simulink model "TRQCTL"  (R2022b)
settings: configuration reference "SharedConfig" (kept outside this file)
values from neighbouring files (symbols this model uses):
  MotTqCon_C = 0.054    [TRQCTL.sldd]
  MotTqGainBdT1_Ax : value not decoded    [TRQCTL.sldd]
  MotTqGainBdT1_T : value not decoded    [TRQCTL.sldd]
  MotTqGainBdT2_Ax : value not decoded    [TRQCTL.sldd]
  MotTqGainBdT2_T : value not decoded    [TRQCTL.sldd]
  MotTqMaxDialEna_C = 0.0    [TRQCTL.sldd]
  MotTqMaxDialVal_C = 0.0    [TRQCTL.sldd]
  MotTqMaxMotSpd_Ax : value not decoded    [TRQCTL.sldd]
  MotTqMaxMotSpd_T : value not decoded    [TRQCTL.sldd]
  PhaCurDTarVal_C = 0.0    [TRQCTL.sldd]
  PhaCurQTarDialEna_C = 1.0    [TRQCTL.sldd]
  PhaCurQTarDialVal_C = 0.0    [TRQCTL.sldd]
undefined symbols (not defined in the file or in its folder): slcm
libraries: simulink x1
Description:
  | Controls the torque of the motor by arbitrating requests and limits and determining phase current targets.
settings Model: DataDictionary=TRQCTL.sldd  Creator=Kevin  LastModifiedBy=Max Kolesnikov
settings ConfigSetRef: SourceName=SharedConfig

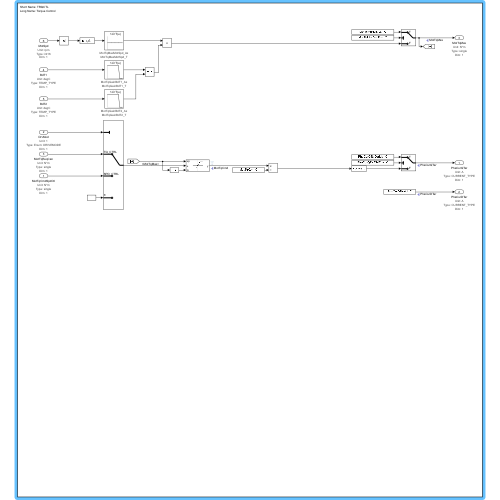
[thumbnail: Simulink's stored preview of the top-level diagram]
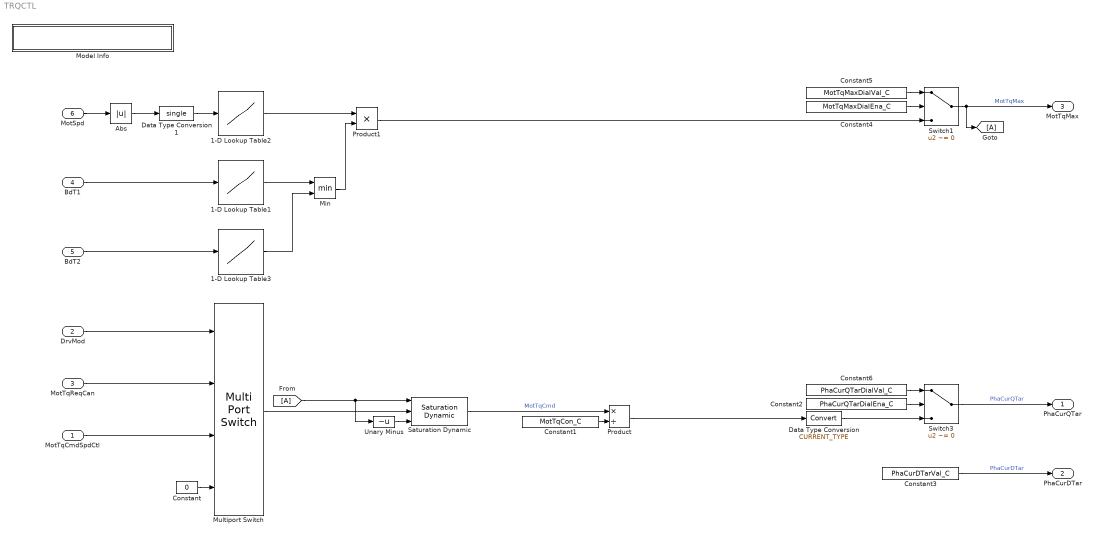
== system TRQCTL ==
  MotTqCmdSpdCtl : Inport  OutDataTypeStr=single  Unit=N*m  PortDimensions=1
      settings: AttributesFormatString=|
      | Unit: %<Unit>
      | Type: %<OutDataTypeStr>
      | Dim: %<PortDimensions>
  DrvMod : Inport  Port=2  OutDataTypeStr=Enum: DRIVEMODE  Unit=1  PortDimensions=1
      settings: AttributesFormatString=|
      | Unit: %<Unit>
      | Type: %<OutDataTypeStr>
      | Dim: %<PortDimensions>
  MotTqReqCan : Inport  Port=3  OutDataTypeStr=single  Unit=N*m  PortDimensions=1
      settings: AttributesFormatString=|
      | Unit: %<Unit>
      | Type: %<OutDataTypeStr>
      | Dim: %<PortDimensions>
  BdT1 : Inport  Port=4  OutDataTypeStr=TEMP_TYPE  Unit=degC  PortDimensions=1
      settings: AttributesFormatString=|
      | Unit: %<Unit>
      | Type: %<OutDataTypeStr>
      | Dim: %<PortDimensions>
  BdT2 : Inport  Port=5  OutDataTypeStr=TEMP_TYPE  Unit=degC  PortDimensions=1
      settings: AttributesFormatString=|
      | Unit: %<Unit>
      | Type: %<OutDataTypeStr>
      | Dim: %<PortDimensions>
  MotSpd : Inport  Port=6  OutDataTypeStr=int16  Unit=rpm  PortDimensions=1
      settings: AttributesFormatString=|
      | Unit: %<Unit>
      | Type: %<OutDataTypeStr>
      | Dim: %<PortDimensions>
  1-D Lookup Table1 : Lookup_n-D  NumberOfTableDimensions=1  BreakpointsForDimension1=MotTqGainBdT1_Ax  Table=MotTqGainBdT1_T  InternalRulePriority=Speed  RndMeth=Simplest
      settings: AttributesFormatString=|
      | %<BreakpointsForDimension1>
      | %<Table>
  1-D Lookup Table2 : Lookup_n-D  NumberOfTableDimensions=1  BreakpointsForDimension1=MotTqMaxMotSpd_Ax  Table=MotTqMaxMotSpd_T  InternalRulePriority=Speed  RndMeth=Simplest
      settings: AttributesFormatString=|
      | %<BreakpointsForDimension1>
      | %<Table>
  1-D Lookup Table3 : Lookup_n-D  NumberOfTableDimensions=1  BreakpointsForDimension1=MotTqGainBdT2_Ax  Table=MotTqGainBdT2_T  InternalRulePriority=Speed  RndMeth=Simplest
      settings: AttributesFormatString=|
      | %<BreakpointsForDimension1>
      | %<Table>
  Abs : Abs  SaturateOnIntegerOverflow=off
  Constant : Constant  Value=0  OutDataTypeStr=single
  Constant1 : Constant  Value=MotTqCon_C
  Constant2 : Constant  Value=PhaCurQTarDialEna_C
  Constant3 : Constant  Value=PhaCurDTarVal_C
  Constant4 : Constant  Value=MotTqMaxDialEna_C
  Constant5 : Constant  Value=MotTqMaxDialVal_C
  Constant6 : Constant  Value=PhaCurQTarDialVal_C
  Data Type Conversion : DataTypeConversion  OutDataTypeStr=CURRENT_TYPE  SaturateOnIntegerOverflow=off  RndMeth=Floor
  Data Type Conversion1 : DataTypeConversion  OutDataTypeStr=single  SaturateOnIntegerOverflow=off  RndMeth=Floor
  From : From
  Goto : Goto
  Min : MinMax  Inputs=2
  Model Info : Subsystem  LoadFcn=slcm LoadBlock;  InitFcn=slcm('UpdateAllCMBlocksInThisModelInit')  mask(CMBlock){Frame=off, DisplayStringWithTags=|, MaskDisplayString=Short Name: TRQCTL\nLong Name: Torque Control, HorizontalTextAlignment=Left, LeftAlignmentValue=0.02}
      mask DisplayStringWithTags=|
      | Short Name: %<ModelName>
      | Long Name: Torque Control
      mask prompts: Frame "Simulink:masks:Frame_MP"; DisplayStringWithTags "Simulink:masks:DisplayStringWithTags_MP"; MaskDisplayString "Simulink:masks:MaskDisplayString_MP"; HorizontalTextAlignment "Simulink:masks:HorizontalTextAlignment_MP"; LeftAlignmentValue "Simulink:masks:LeftAlignmentValue_MP"
      mask help: Simulink:masks:CMBlock_MD
      settings: CopyFcn=slcm CopyBlock;  DeleteFcn=slcm Cancel;  PostSaveFcn=slcm('UpdateAllCMBlocksInThisModel')  NameChangeFcn=slcm Rename;  OpenFcn=slcm
      mask Display: text(slResolve(LeftAlignmentValue, gcbh), 0.5, MaskDisplayString, 'HorizontalAlignment', HorizontalTextAlignment)
  Multiport Switch : MultiPortSwitch  DataPortOrder=Specify indices  DataPortIndices={DRIVEMODE.TQ_CTRL,DRIVEMODE.SPD_CTRL}  DataPortForDefault=Additional data port  DiagnosticForDefault=None  SaturateOnIntegerOverflow=off  InputSameDT=off
  Product : Product  Inputs=*/
  Product1 : Product
  Saturation Dynamic : simulink/Discontinuities/Saturation Dynamic  OutMin=[]  OutMax=[]  OutDataTypeStr=Inherit: Same as second input  OutDataType=fixdt(1, 16)  OutScaling=2^-10  DoSatur=off
  Switch1 : Switch  Criteria=u2 ~= 0  SaturateOnIntegerOverflow=off  InputSameDT=off
  Switch3 : Switch  Criteria=u2 ~= 0  SaturateOnIntegerOverflow=off  InputSameDT=off
  Unary Minus : UnaryMinus
  PhaCurQTar : Outport  OutDataTypeStr=CURRENT_TYPE  Unit=A  PortDimensions=1
      settings: AttributesFormatString=|
      | Unit: %<Unit>
      | Type: %<OutDataTypeStr>
      | Dim: %<PortDimensions>
  PhaCurDTar : Outport  Port=2  OutDataTypeStr=CURRENT_TYPE  Unit=A  PortDimensions=1
      settings: AttributesFormatString=|
      | Unit: %<Unit>
      | Type: %<OutDataTypeStr>
      | Dim: %<PortDimensions>
  MotTqMax : Outport  Port=3  OutDataTypeStr=single  Unit=N*m  PortDimensions=1
      settings: AttributesFormatString=|
      | Unit: %<Unit>
      | Type: %<OutDataTypeStr>
      | Dim: %<PortDimensions>
  wires:
  DrvMod/1 -> Multiport Switch/1
  MotTqCmdSpdCtl/1 -> Multiport Switch/3
  Constant/1 -> Multiport Switch/4
  Constant1/1 -> Product/2
  Product/1 -> Data Type Conversion/1
  Constant3/1 -> PhaCurDTar/1  "PhaCurDTar"
  Multiport Switch/1 -> Saturation Dynamic/2
  Switch3/1 -> PhaCurQTar/1  "PhaCurQTar"
  MotTqReqCan/1 -> Multiport Switch/2
  Constant6/1 -> Switch3/1
  Constant2/1 -> Switch3/2
  Data Type Conversion/1 -> Switch3/3
  Constant4/1 -> Switch1/2
  Constant5/1 -> Switch1/1
  Switch1/1 -> Goto/1, MotTqMax/1  "MotTqMax"
  BdT2/1 -> 1-D Lookup Table3/1
  BdT1/1 -> 1-D Lookup Table1/1
  1-D Lookup Table1/1 -> Min/1
  1-D Lookup Table3/1 -> Min/2
  MotSpd/1 -> Abs/1
  1-D Lookup Table2/1 -> Product1/1
  Min/1 -> Product1/2
  Product1/1 -> Switch1/3
  Saturation Dynamic/1 -> Product/1  "MotTqCmd"
  Unary Minus/1 -> Saturation Dynamic/3
  From/1 -> Saturation Dynamic/1, Unary Minus/1
  Abs/1 -> Data Type Conversion1/1
  Data Type Conversion1/1 -> 1-D Lookup Table2/1

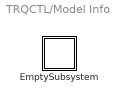
== system TRQCTL/Model Info ==
  EmptySubsystem : Subsystem

== system TRQCTL/Model Info/EmptySubsystem ==
